simulink model "pose_control"  (R2025b)
settings: Solver=FixedStepAuto  StartTime=0.0  StopTime=t_end  FixedStep=dt  RelTol=1e-3
undefined symbols (not defined in the file or in its folder): kg, p_init, p_r, theta_init, theta_r
settings Model: Creator=yamauchi  LastModifiedBy=tanabe

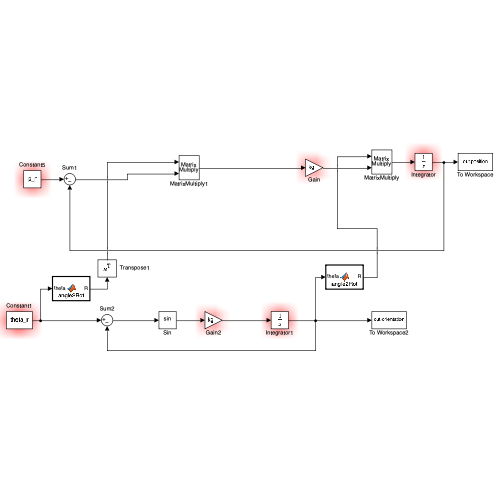
[thumbnail: Simulink's stored preview of the top-level diagram]
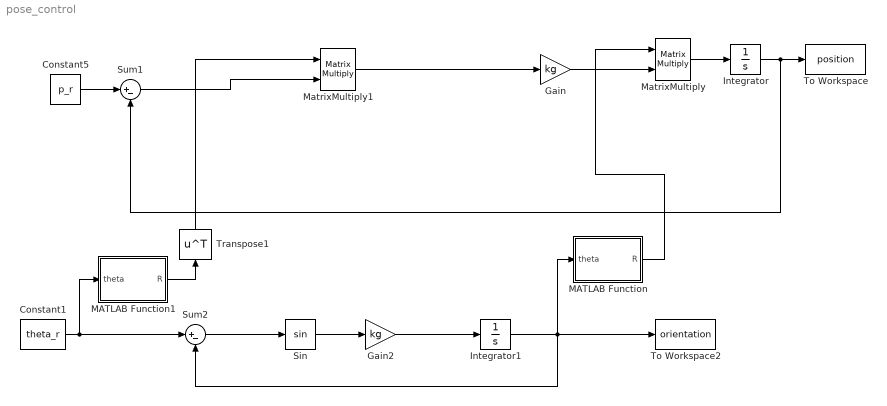
== system pose_control ==
  Constant1 : Constant  Value=theta_r
  Constant5 : Constant  Value=p_r
  Gain : Gain  Gain=kg
  Gain2 : Gain  Gain=kg
  Integrator : Integrator  InitialCondition=p_init
  Integrator1 : Integrator  InitialCondition=theta_init
  MATLAB Function : MATLAB Function  TreatAsAtomicUnit=on
  MATLAB Function1 : MATLAB Function  TreatAsAtomicUnit=on
  MatrixMultiply : Product  Multiplication=Matrix(*)
  MatrixMultiply1 : Product  Multiplication=Matrix(*)
  Sin : Trigonometry
  Sum1 : Sum  Inputs=|+-
  Sum2 : Sum  Inputs=|+-
  To Workspace : ToWorkspace  VariableName=position  SampleTime=-1
      settings: Save2DSignal=2-D array (concatenate along first dimension)
  To Workspace2 : ToWorkspace  VariableName=orientation  SampleTime=-1
      settings: Save2DSignal=2-D array (concatenate along first dimension)
  Transpose1 : Math  Operator=transpose
  wires:
  Integrator1/1 -> To Workspace2/1, MATLAB Function/1(theta), Sum2/2
  Integrator/1 -> To Workspace/1, Sum1/2
  MatrixMultiply/1 -> Integrator/1
  Gain/1 -> MatrixMultiply/2
  Gain2/1 -> Integrator1/1
  Sin/1 -> Gain2/1
  Constant1/1 -> Sum2/1, MATLAB Function1/1(theta)
  Sum2/1 -> Sin/1
  Constant5/1 -> Sum1/1
  MATLAB Function/1(R) -> MatrixMultiply/1
  MATLAB Function1/1(R) -> Transpose1/1
  Transpose1/1 -> MatrixMultiply1/1
  Sum1/1 -> MatrixMultiply1/2
  MatrixMultiply1/1 -> Gain/1

== matlab function pose_control/MATLAB Function ==
  data: theta input; R output
function R = angle2Rot(theta)

R = [cos(theta) -sin(theta); sin(theta) cos(theta)];

== matlab function pose_control/MATLAB Function1 ==
  data: theta input; R output
function R = angle2Rot(theta)

R = [cos(theta) -sin(theta); sin(theta) cos(theta)];
